simulink model "six_plus_six_AcmsteeringV09_main"  (R2014a)
settings: Solver=FixedStepDiscrete  StartTime=0.0  StopTime=10.0  FixedStep=0.0005  RelTol=1e-3
InitFcn:
  | Veh_Par_wxt
values from neighbouring files (symbols this model uses):
  acc_spdctl = [0 100]    [Veh_Par_wxt.m]
  ag_thr = ecucoder_cal(ag_thr)    [Veh_Par_wxt.m]
  B = 1.8    [Veh_Par_wxt.m]
  bra_em = 100    [Veh_Par_wxt.m]
  bra_pre_gz2 = 100/3    (= 33.3333333333)    [Veh_Par_wxt.m]
  bra_pre_gz34 = 10/3    (= 3.33333333333)    [Veh_Par_wxt.m]
  bra_pre_yd = 10/2    (= 5)    [Veh_Par_wxt.m]
  brakepre_dem_data = [0 1 2 3 4 5 6 7 8 9 10]    [Veh_Par_wxt.m]
  brakeTrq_dem_data = [0 125 251 376 502 627 753 878 1004 1129 1255]    [Veh_Par_wxt.m]
  bratrq_max = 4*1255    (= 5020)    [Veh_Par_wxt.m]
  eff_tran = 0.9    [Veh_Par_wxt.m]
  ESP_switch = ecucoder_cal(ESP_switch)    [Veh_Par_wxt.m]
  G = Mass*g    (= 15696)    [Veh_Par_wxt.m]
  kd1 = ecucoder_cal(kd1)    [Veh_Par_wxt.m]
  kd2 = 0    [Veh_Par_wxt.m]
  ki1 = ecucoder_cal(ki1)    [Veh_Par_wxt.m]
  ki2 = 1    [Veh_Par_wxt.m]
  kp1 = ecucoder_cal(kp1)    [Veh_Par_wxt.m]
  kp2 = 300    [Veh_Par_wxt.m]
  L = L1+L2    (= 2.9)    [Veh_Par_wxt.m]
  premax = 100    [Veh_Par_wxt.m]
  Radius = 0.4572/2    (= 0.2286)    [Veh_Par_wxt.m]
  RC_switch = ecucoder_cal(RC_switch)    [Veh_Par_wxt.m]
  s_opt_yi = 0.15    [Veh_Par_wxt.m]
  s_opt_zhuan = 0.8    [Veh_Par_wxt.m]
  s_opt_zhuan_add = 0.05    [Veh_Par_wxt.m]
  s_opt_zhuan_table = [0.8 0.8 0.3 0.3]    [Veh_Par_wxt.m]
  spd_map_mot = [0 499.85 999.79 1500 2000 2500 3000 3500 4000 4500 4999.8 5999.8]    [Veh_Par_wxt.m]
  spd_spdctl = [0 500]    [Veh_Par_wxt.m]
  speed_thr_park = 5/3.6/Radius*tras_ratio*30/pi    (= 464.143899364)    [Veh_Par_wxt.m]
  TCS_switch = ecucoder_cal(TCS_switch)    [Veh_Par_wxt.m]
  tras_ratio = 8    [Veh_Par_wxt.m]
  trq_map_mot = [70.5 70.012 71.154 65.797 53.917 45.159 38.073 32.685 27.48 17.133 14.949 10.07]    [Veh_Par_wxt.m]
  trqmax_yd = 70.5    [Veh_Par_wxt.m]
  trqmax_zx = 70.5    [Veh_Par_wxt.m]
  trqmaxneg = -70.5    [Veh_Par_wxt.m]
  v_gain = 0.9    [Veh_Par_wxt.m]
  v_table = [0 5 20 100]    [Veh_Par_wxt.m]
  v_thr_park = 5    [Veh_Par_wxt.m]
  zhidong_bianmazhi = [-140000 750000]    [Veh_Par_wxt.m]
  zhidong_down = -140000    [Veh_Par_wxt.m]
  zhidong_up = 750000    [Veh_Par_wxt.m]
  zhidong_youmen = [0 100]    [Veh_Par_wxt.m]
  zhuanxiang_bianmazhi = [-400000 0 400000]    [Veh_Par_wxt.m]
  zhuanxiang_down = -400000    [Veh_Par_wxt.m]
  zhuanxiang_up = 400000    [Veh_Par_wxt.m]
  zhuanxiang_youmen = [-100 0 100]    [Veh_Par_wxt.m]
undefined symbols (not defined in the file or in its folder): ecucoder_acal, guzhang_lf, guzhang_lm, guzhang_lr, guzhang_rf, guzhang_rm, guzhang_rr, myFIS
libraries: simulink x979, ec5744lib x59, fuzblock x2
(part 8 of 26)

== system six_plus_six_AcmsteeringV09_main/Data_input/MCU0_4/MCU0 ==
  input : Inport
  Enable : EnablePort
  Demux : Demux  Outputs=8
  MCU0_ControlMode_Ad : Sum
  MCU0_ControlMode_Convert : DataTypeConversion  OutDataTypeStr=uint32
  MCU0_ControlMode_F : Gain
  MCU0_ControlMode_L : simulink/Logic and Bit Operations/Bitwise Operator  logicop=AND  UseBitMask=on  BitMask=4  BitMaskRealWorld=Stored Integer
  MCU0_ControlMode_O : Constant  Value=0  OutDataTypeStr=single
  MCU0_ControlMode_S : ArithShift  BitShiftNumber=2
  MCU0_ControlMode_Sub : Subsystem
  MCU0_ControlMode_sat : Saturate  UpperLimit=1  LowerLimit=0
  MCU0_ControlModecv : DataTypeConversion
  MCU0_EmergShutDown_Ad : Sum
  MCU0_EmergShutDown_Convert : DataTypeConversion  OutDataTypeStr=uint32
  MCU0_EmergShutDown_F : Gain
  MCU0_EmergShutDown_L : simulink/Logic and Bit Operations/Bitwise Operator  logicop=AND  UseBitMask=on  BitMask=128  BitMaskRealWorld=Stored Integer
  MCU0_EmergShutDown_O : Constant  Value=0  OutDataTypeStr=single
  MCU0_EmergShutDown_S : ArithShift  BitShiftNumber=7
  MCU0_EmergShutDown_Sub : Subsystem
  MCU0_EmergShutDown_sat : Saturate  UpperLimit=1  LowerLimit=0
  MCU0_EmergShutDowncv : DataTypeConversion
  MCU0_GearStatus_Ad : Sum
  MCU0_GearStatus_Convert : DataTypeConversion  OutDataTypeStr=uint32
  MCU0_GearStatus_F : Gain
  MCU0_GearStatus_L : simulink/Logic and Bit Operations/Bitwise Operator  logicop=AND  UseBitMask=on  BitMask=24  BitMaskRealWorld=Stored Integer
  MCU0_GearStatus_O : Constant  Value=0  OutDataTypeStr=single
  MCU0_GearStatus_S : ArithShift  BitShiftNumber=3
  MCU0_GearStatus_Sub : Subsystem
  MCU0_GearStatus_sat : Saturate  UpperLimit=3  LowerLimit=0
  MCU0_GearStatuscv : DataTypeConversion
  MCU0_HighVol_Ad : Sum
  MCU0_HighVol_Convert : DataTypeConversion  OutDataTypeStr=uint32
  MCU0_HighVol_F : Gain
  MCU0_HighVol_L : simulink/Logic and Bit Operations/Bitwise Operator  logicop=AND  UseBitMask=on  BitMask=32  BitMaskRealWorld=Stored Integer
  MCU0_HighVol_O : Constant  Value=0  OutDataTypeStr=single
  MCU0_HighVol_S : ArithShift  BitShiftNumber=5
  MCU0_HighVol_Sub : Subsystem
  MCU0_HighVol_sat : Saturate  UpperLimit=1  LowerLimit=0
  MCU0_HighVolcv : DataTypeConversion
  MCU0_LiftCnt_Ad : Sum
  MCU0_LiftCnt_Convert : DataTypeConversion  OutDataTypeStr=uint32
  MCU0_LiftCnt_F : Gain
  MCU0_LiftCnt_L : simulink/Logic and Bit Operations/Bitwise Operator  logicop=AND  UseBitMask=on  BitMask=255  BitMaskRealWorld=Stored Integer
  MCU0_LiftCnt_O : Constant  Value=0  OutDataTypeStr=single
  MCU0_LiftCnt_S : ArithShift
  MCU0_LiftCnt_Sub : Subsystem
  MCU0_LiftCnt_sat : Saturate  UpperLimit=255  LowerLimit=0
  MCU0_LiftCntcv : DataTypeConversion
  MCU0_ShutDowAllow_Ad : Sum
  MCU0_ShutDowAllow_Convert : DataTypeConversion  OutDataTypeStr=uint32
  MCU0_ShutDowAllow_F : Gain
  MCU0_ShutDowAllow_L : simulink/Logic and Bit Operations/Bitwise Operator  logicop=AND  UseBitMask=on  BitMask=64  BitMaskRealWorld=Stored Integer
  MCU0_ShutDowAllow_O : Constant  Value=0  OutDataTypeStr=single
  MCU0_ShutDowAllow_S : ArithShift  BitShiftNumber=6
  MCU0_ShutDowAllow_Sub : Subsystem
  MCU0_ShutDowAllow_sat : Saturate  UpperLimit=1  LowerLimit=0
  MCU0_ShutDowAllowcv : DataTypeConversion
  MCU0_SpeedFdk_Ad : Sum
  MCU0_SpeedFdk_Convert : DataTypeConversion  OutDataTypeStr=uint32
  MCU0_SpeedFdk_F : Gain
  MCU0_SpeedFdk_L : simulink/Logic and Bit Operations/Bitwise Operator  logicop=AND  UseBitMask=on  BitMask=65535  BitMaskRealWorld=Stored Integer
  MCU0_SpeedFdk_O : Constant  Value=-10000  OutDataTypeStr=single
  MCU0_SpeedFdk_S : ArithShift
  MCU0_SpeedFdk_Sub : Subsystem
  MCU0_SpeedFdk_sat : Saturate  UpperLimit=10000  LowerLimit=-10000
  MCU0_SpeedFdkcv : DataTypeConversion
  MCU0_SpeedFdkinput2_Ad : Sum
  MCU0_SpeedFdkinput2_C : Constant  Value=256
  MCU0_SpeedFdkinput2_P : Product
  MCU0_TorqueFdk_Ad : Sum
  MCU0_TorqueFdk_Convert : DataTypeConversion  OutDataTypeStr=uint32
  MCU0_TorqueFdk_F : Gain  Gain=0.1
  MCU0_TorqueFdk_L : simulink/Logic and Bit Operations/Bitwise Operator  logicop=AND  UseBitMask=on  BitMask=65535  BitMaskRealWorld=Stored Integer
  MCU0_TorqueFdk_O : Constant  Value=-1000  OutDataTypeStr=single
  MCU0_TorqueFdk_S : ArithShift
  MCU0_TorqueFdk_Sub : Subsystem
  MCU0_TorqueFdk_sat : Saturate  UpperLimit=1000  LowerLimit=-1000
  MCU0_TorqueFdkcv : DataTypeConversion
  MCU0_TorqueFdkinput4_Ad : Sum
  MCU0_TorqueFdkinput4_C : Constant  Value=256
  MCU0_TorqueFdkinput4_P : Product
  MCU0_TorqueMax_Ad : Sum
  MCU0_TorqueMax_Convert : DataTypeConversion  OutDataTypeStr=uint32
  MCU0_TorqueMax_F : Gain  Gain=0.1
  MCU0_TorqueMax_L : simulink/Logic and Bit Operations/Bitwise Operator  logicop=AND  UseBitMask=on  BitMask=65535  BitMaskRealWorld=Stored Integer
  MCU0_TorqueMax_O : Constant  Value=-1000  OutDataTypeStr=single
  MCU0_TorqueMax_S : ArithShift
  MCU0_TorqueMax_Sub : Subsystem
  MCU0_TorqueMax_sat : Saturate  UpperLimit=1000  LowerLimit=-1000
  MCU0_TorqueMaxcv : DataTypeConversion
  MCU0_TorqueMaxinput6_Ad : Sum
  MCU0_TorqueMaxinput6_C : Constant  Value=256
  MCU0_TorqueMaxinput6_P : Product
  MCU0_WorkStatus_Ad : Sum
  MCU0_WorkStatus_Convert : DataTypeConversion  OutDataTypeStr=uint32
  MCU0_WorkStatus_F : Gain
  MCU0_WorkStatus_L : simulink/Logic and Bit Operations/Bitwise Operator  logicop=AND  UseBitMask=on  BitMask=3  BitMaskRealWorld=Stored Integer
  MCU0_WorkStatus_O : Constant  Value=0  OutDataTypeStr=single
  MCU0_WorkStatus_S : ArithShift
  MCU0_WorkStatus_Sub : Subsystem
  MCU0_WorkStatus_sat : Saturate  UpperLimit=3  LowerLimit=0
  MCU0_WorkStatuscv : DataTypeConversion
  MCU0_TorqueMax_Out : Outport
  MCU0_EmergShutDown_Out : Outport  Port=2
  MCU0_ShutDowAllow_Out : Outport  Port=3
  MCU0_HighVol_Out : Outport  Port=4
  MCU0_LiftCnt_Out : Outport  Port=5
  MCU0_TorqueFdk_Out : Outport  Port=6
  MCU0_SpeedFdk_Out : Outport  Port=7
  MCU0_GearStatus_Out : Outport  Port=8
  MCU0_ControlMode_Out : Outport  Port=9
  MCU0_WorkStatus_Out : Outport  Port=10
  wires:
  MCU0_TorqueMax_F/1 -> MCU0_TorqueMax_Ad/1
  MCU0_TorqueMax_O/1 -> MCU0_TorqueMax_Ad/2
  MCU0_TorqueMax_Ad/1 -> MCU0_TorqueMax_sat/1
  MCU0_TorqueMax_sat/1 -> MCU0_TorqueMax_Out/1
  Demux/6 -> MCU0_TorqueMaxinput6_P/1
  MCU0_TorqueMaxinput6_C/1 -> MCU0_TorqueMaxinput6_P/2
  MCU0_TorqueMaxinput6_P/1 -> MCU0_TorqueMaxinput6_Ad/1
  Demux/7 -> MCU0_TorqueMaxinput6_Ad/2
  MCU0_TorqueMaxinput6_Ad/1 -> MCU0_TorqueMax_Sub/1(In1)
  MCU0_TorqueMax_Sub/1(Out1) -> MCU0_TorqueMax_Convert/1
  MCU0_TorqueMax_Convert/1 -> MCU0_TorqueMax_L/1
  MCU0_TorqueMax_L/1 -> MCU0_TorqueMax_S/1
  MCU0_TorqueMax_S/1 -> MCU0_TorqueMaxcv/1
  MCU0_TorqueMaxcv/1 -> MCU0_TorqueMax_F/1
  MCU0_EmergShutDown_F/1 -> MCU0_EmergShutDown_Ad/1
  MCU0_EmergShutDown_O/1 -> MCU0_EmergShutDown_Ad/2
  MCU0_EmergShutDown_Ad/1 -> MCU0_EmergShutDown_sat/1
  MCU0_EmergShutDown_sat/1 -> MCU0_EmergShutDown_Out/1
  Demux/1 -> MCU0_ControlMode_Sub/1(In1), MCU0_WorkStatus_Sub/1(In1), MCU0_GearStatus_Sub/1(In1), MCU0_HighVol_Sub/1(In1), MCU0_ShutDowAllow_Sub/1(In1), MCU0_EmergShutDown_Sub/1(In1)
  MCU0_EmergShutDown_Sub/1(Out1) -> MCU0_EmergShutDown_Convert/1
  MCU0_EmergShutDown_Convert/1 -> MCU0_EmergShutDown_L/1
  MCU0_EmergShutDown_L/1 -> MCU0_EmergShutDown_S/1
  MCU0_EmergShutDown_S/1 -> MCU0_EmergShutDowncv/1
  MCU0_EmergShutDowncv/1 -> MCU0_EmergShutDown_F/1
  MCU0_ShutDowAllow_F/1 -> MCU0_ShutDowAllow_Ad/1
  MCU0_ShutDowAllow_O/1 -> MCU0_ShutDowAllow_Ad/2
  MCU0_ShutDowAllow_Ad/1 -> MCU0_ShutDowAllow_sat/1
  MCU0_ShutDowAllow_sat/1 -> MCU0_ShutDowAllow_Out/1
  MCU0_ShutDowAllow_Sub/1(Out1) -> MCU0_ShutDowAllow_Convert/1
  MCU0_ShutDowAllow_Convert/1 -> MCU0_ShutDowAllow_L/1
  MCU0_ShutDowAllow_L/1 -> MCU0_ShutDowAllow_S/1
  MCU0_ShutDowAllow_S/1 -> MCU0_ShutDowAllowcv/1
  MCU0_ShutDowAllowcv/1 -> MCU0_ShutDowAllow_F/1
  MCU0_HighVol_F/1 -> MCU0_HighVol_Ad/1
  MCU0_HighVol_O/1 -> MCU0_HighVol_Ad/2
  MCU0_HighVol_Ad/1 -> MCU0_HighVol_sat/1
  MCU0_HighVol_sat/1 -> MCU0_HighVol_Out/1
  MCU0_HighVol_Sub/1(Out1) -> MCU0_HighVol_Convert/1
  MCU0_HighVol_Convert/1 -> MCU0_HighVol_L/1
  MCU0_HighVol_L/1 -> MCU0_HighVol_S/1
  MCU0_HighVol_S/1 -> MCU0_HighVolcv/1
  MCU0_HighVolcv/1 -> MCU0_HighVol_F/1
  MCU0_LiftCnt_F/1 -> MCU0_LiftCnt_Ad/1
  MCU0_LiftCnt_O/1 -> MCU0_LiftCnt_Ad/2
  MCU0_LiftCnt_Ad/1 -> MCU0_LiftCnt_sat/1
  MCU0_LiftCnt_sat/1 -> MCU0_LiftCnt_Out/1
  Demux/8 -> MCU0_LiftCnt_Sub/1(In1)
  MCU0_LiftCnt_Sub/1(Out1) -> MCU0_LiftCnt_Convert/1
  MCU0_LiftCnt_Convert/1 -> MCU0_LiftCnt_L/1
  MCU0_LiftCnt_L/1 -> MCU0_LiftCnt_S/1
  MCU0_LiftCnt_S/1 -> MCU0_LiftCntcv/1
  MCU0_LiftCntcv/1 -> MCU0_LiftCnt_F/1
  MCU0_TorqueFdk_F/1 -> MCU0_TorqueFdk_Ad/1
  MCU0_TorqueFdk_O/1 -> MCU0_TorqueFdk_Ad/2
  MCU0_TorqueFdk_Ad/1 -> MCU0_TorqueFdk_sat/1
  MCU0_TorqueFdk_sat/1 -> MCU0_TorqueFdk_Out/1
  Demux/4 -> MCU0_TorqueFdkinput4_P/1
  MCU0_TorqueFdkinput4_C/1 -> MCU0_TorqueFdkinput4_P/2
  MCU0_TorqueFdkinput4_P/1 -> MCU0_TorqueFdkinput4_Ad/1
  Demux/5 -> MCU0_TorqueFdkinput4_Ad/2
  MCU0_TorqueFdkinput4_Ad/1 -> MCU0_TorqueFdk_Sub/1(In1)
  MCU0_TorqueFdk_Sub/1(Out1) -> MCU0_TorqueFdk_Convert/1
  MCU0_TorqueFdk_Convert/1 -> MCU0_TorqueFdk_L/1
  MCU0_TorqueFdk_L/1 -> MCU0_TorqueFdk_S/1
  MCU0_TorqueFdk_S/1 -> MCU0_TorqueFdkcv/1
  MCU0_TorqueFdkcv/1 -> MCU0_TorqueFdk_F/1
  MCU0_SpeedFdk_F/1 -> MCU0_SpeedFdk_Ad/1
  MCU0_SpeedFdk_O/1 -> MCU0_SpeedFdk_Ad/2
  MCU0_SpeedFdk_Ad/1 -> MCU0_SpeedFdk_sat/1
  MCU0_SpeedFdk_sat/1 -> MCU0_SpeedFdk_Out/1
  Demux/2 -> MCU0_SpeedFdkinput2_P/1
  MCU0_SpeedFdkinput2_C/1 -> MCU0_SpeedFdkinput2_P/2
  MCU0_SpeedFdkinput2_P/1 -> MCU0_SpeedFdkinput2_Ad/1
  Demux/3 -> MCU0_SpeedFdkinput2_Ad/2
  MCU0_SpeedFdkinput2_Ad/1 -> MCU0_SpeedFdk_Sub/1(In1)
  MCU0_SpeedFdk_Sub/1(Out1) -> MCU0_SpeedFdk_Convert/1
  MCU0_SpeedFdk_Convert/1 -> MCU0_SpeedFdk_L/1
  MCU0_SpeedFdk_L/1 -> MCU0_SpeedFdk_S/1
  MCU0_SpeedFdk_S/1 -> MCU0_SpeedFdkcv/1
  MCU0_SpeedFdkcv/1 -> MCU0_SpeedFdk_F/1
  MCU0_GearStatus_F/1 -> MCU0_GearStatus_Ad/1
  MCU0_GearStatus_O/1 -> MCU0_GearStatus_Ad/2
  MCU0_GearStatus_Ad/1 -> MCU0_GearStatus_sat/1
  MCU0_GearStatus_sat/1 -> MCU0_GearStatus_Out/1
  MCU0_GearStatus_Sub/1(Out1) -> MCU0_GearStatus_Convert/1
  MCU0_GearStatus_Convert/1 -> MCU0_GearStatus_L/1
  MCU0_GearStatus_L/1 -> MCU0_GearStatus_S/1
  MCU0_GearStatus_S/1 -> MCU0_GearStatuscv/1
  MCU0_GearStatuscv/1 -> MCU0_GearStatus_F/1
  MCU0_ControlMode_F/1 -> MCU0_ControlMode_Ad/1
  MCU0_ControlMode_O/1 -> MCU0_ControlMode_Ad/2
  MCU0_ControlMode_Ad/1 -> MCU0_ControlMode_sat/1
  MCU0_ControlMode_sat/1 -> MCU0_ControlMode_Out/1
  MCU0_ControlMode_Sub/1(Out1) -> MCU0_ControlMode_Convert/1
  MCU0_ControlMode_Convert/1 -> MCU0_ControlMode_L/1
  MCU0_ControlMode_L/1 -> MCU0_ControlMode_S/1
  MCU0_ControlMode_S/1 -> MCU0_ControlModecv/1
  MCU0_ControlModecv/1 -> MCU0_ControlMode_F/1
  MCU0_WorkStatus_F/1 -> MCU0_WorkStatus_Ad/1
  MCU0_WorkStatus_O/1 -> MCU0_WorkStatus_Ad/2
  MCU0_WorkStatus_Ad/1 -> MCU0_WorkStatus_sat/1
  MCU0_WorkStatus_sat/1 -> MCU0_WorkStatus_Out/1
  MCU0_WorkStatus_Sub/1(Out1) -> MCU0_WorkStatus_Convert/1
  MCU0_WorkStatus_Convert/1 -> MCU0_WorkStatus_L/1
  MCU0_WorkStatus_L/1 -> MCU0_WorkStatus_S/1
  MCU0_WorkStatus_S/1 -> MCU0_WorkStatuscv/1
  MCU0_WorkStatuscv/1 -> MCU0_WorkStatus_F/1
  input/1 -> Demux/1

== matlab function six_plus_six_AcmsteeringV09_main/MainControl/mode_control/forward/forward/Brake/HeartBeat5 ==
  data: life_pre input; life output
function life = fcn(life_pre)
%#codegen
life=single(life_pre+1);
if life>255
    life=single(0);
end
end

== matlab function six_plus_six_AcmsteeringV09_main/MainControl/mode_control/neutral/neutral/HeartBeat2 ==
  data: life_pre input; life output
function life = fcn(life_pre)
%#codegen
life=single(life_pre+1);
if life>255
    life=single(0);
end
end

== matlab function six_plus_six_AcmsteeringV09_main/MainControl/mode_control/backward/backward/Brake/HeartBeat4 ==
  data: life_pre input; life output
function life = fcn(life_pre)
%#codegen
life=single(life_pre+1);
if life>255
    life=single(0);
end
end

== matlab function six_plus_six_AcmsteeringV09_main/MainControl/mode_control/backward/backward/Drive/目标转向力矩确定模块/MATLAB Function1 ==
  data: v_act input; Rturn_min_ag output; ag_thr input
 function Rturn_min_ag = fcn(v_act,ag_thr)
%#codegen

    Rturn_min_ag=single((v_act/3.6)^2/ag_thr);
end

== matlab function six_plus_six_AcmsteeringV09_main/MainControl/mode_control/backward/backward/Drive/驱动防滑控制TCS/直行TCS/直行/HeartBeat ==
  data: life_pre input; life output
function life = fcn(life_pre)
%#codegen
life=single(life_pre+1);
if life>255
    life=single(0);
end
end

== matlab function six_plus_six_AcmsteeringV09_main/MainControl/mode_control/backward/backward/Drive/驱动防滑控制TCS/直行TCS/直行/HeartBeat2 ==
  data: life_pre input; life output
function life = fcn(life_pre)
%#codegen
life=single(life_pre+1);
if life>255
    life=single(0);
end
end

== matlab function six_plus_six_AcmsteeringV09_main/MainControl/mode_control/backward/backward/MATLAB Function ==
  data: acc_dem input; y output; brake_dem input; HAC input
function y = fcn(acc_dem,brake_dem,HAC)
%#codegen
if HAC==1
    if acc_dem<0
        y=int8(0);
    else
        y=int8(1);
    end
else
    if brake_dem==0
        y=int8(0);
    else
        y=int8(1);
    end
end
end

== matlab function six_plus_six_AcmsteeringV09_main/MainControl/mode_control/emergency_stop/emergency_stop/HeartBeat1 ==
  data: life_pre input; life output
function life = fcn(life_pre)
%#codegen
life=single(life_pre+1);
if life>255
    life=single(0);
end
end

== matlab function six_plus_six_AcmsteeringV09_main/Data_input/1/Enabled
Subsystem/MATLAB Function1 ==
  data: current_in input; current_out output
function current_out = motec_current(current_in)
    if current_in>32768
        current_out=current_in-65535;
    else
        current_out=current_in;
    end
end

== matlab function six_plus_six_AcmsteeringV09_main/MainControl/mode_control/forward/forward/Drive/驱动防滑控制TCS/直行TCS/直行/MATLAB Function6 ==
  data: s_act_rm input; flag_rm output; s_opt_zhuan input; s_opt_zhuan_add input; flag_rm_pre input int8
function flag_rm = fcn(s_act_rm,s_opt_zhuan,s_opt_zhuan_add,flag_rm_pre)
%#codegen
if s_act_rm>s_opt_zhuan+s_opt_zhuan_add
    flag_rm=int8(1);
elseif s_act_rm<s_opt_zhuan
    flag_rm =int8(0);
else
    flag_rm=int8(flag_rm_pre);
end
end

== matlab function six_plus_six_AcmsteeringV09_main/Data_input/4/Enabled Subsystem/MATLAB Function ==
  data: data1 input; y output; data2 input; data3 input; data4 input
function y = fcn(data1,data2,data3,data4)
%#codegen
y1=data4*256^3+data3*256^2+data2*256+data1;
y=typecast(uint32(y1),'single');
end
% y = u;

== matlab function six_plus_six_AcmsteeringV09_main/Data_input/6/Enabled
Subsystem/MATLAB Function1 ==
  data: data1 input; y output; data2 input; data3 input; data4 input
function y = fcn(data1,data2,data3,data4)
%#codegen
y1=data4*256^3+data3*256^2+data2*256+data1;
y=typecast(uint32(y1),'single');
end
% y = u;

== matlab function six_plus_six_AcmsteeringV09_main/Data_input/10/Enabled Subsystem/MATLAB Function ==
  data: data1 input; y output; data2 input; data3 input; data4 input
function y = fcn(data1,data2,data3,data4)
%#codegen
y1=data4*256^3+data3*256^2+data2*256+data1;
y=typecast(uint32(y1),'single');
end
% y = u;

== matlab function six_plus_six_AcmsteeringV09_main/MainControl/mode_control/forward/forward/Drive/MATLAB Function ==
  data: acc_y input; y output; ag_thr input
function y = fcn(acc_y,ag_thr)
%#codegen
if abs(acc_y)>=ag_thr
    y=int8(0);
else 
    y=int8(1);
end
end

== matlab function six_plus_six_AcmsteeringV09_main/MainControl/mode_control/forward/forward/Drive/驱动防滑控制TCS/直行TCS/直行/MATLAB Function5 ==
  data: TCS_switch input; flag_lf1 output; flag_lm1 output; flag_lf input; flag_lm input; flag_lr input; flag_lr1 output; flag_rf input; flag_rm input; flag_rr input; flag_rf1 output; flag_rm1 output; flag_rr1 output
 function [flag_lf1,flag_lm1,flag_lr1,flag_rf1,flag_rm1,flag_rr1] = fcn(TCS_switch,flag_lf,flag_lm,flag_lr,flag_rf,flag_rm,flag_rr)
%#codegen
if TCS_switch==0
    flag_lf1=single(0);
    flag_lm1=single(0);
    flag_lr1=single(0);
    flag_rf1=single(0);
    flag_rm1=single(0);
    flag_rr1=single(0);
else
    flag_lf1=single(flag_lf);
    flag_lm1=single(flag_lm);
    flag_lr1=single(flag_lr);
    flag_rf1=single(flag_rf);
    flag_rm1=single(flag_rm);
    flag_rr1=single(flag_rr);
end
end

== system six_plus_six_AcmsteeringV09_main/Data_input/MCU0_5/MCU0 ==
  input : Inport
  Enable : EnablePort
  Demux : Demux  Outputs=8
  MCU0_ControlMode_Ad : Sum
  MCU0_ControlMode_Convert : DataTypeConversion  OutDataTypeStr=uint32
  MCU0_ControlMode_F : Gain
  MCU0_ControlMode_L : simulink/Logic and Bit Operations/Bitwise Operator  logicop=AND  UseBitMask=on  BitMask=4  BitMaskRealWorld=Stored Integer
  MCU0_ControlMode_O : Constant  Value=0  OutDataTypeStr=single
  MCU0_ControlMode_S : ArithShift  BitShiftNumber=2
  MCU0_ControlMode_Sub : Subsystem
  MCU0_ControlMode_sat : Saturate  UpperLimit=1  LowerLimit=0
  MCU0_ControlModecv : DataTypeConversion
  MCU0_EmergShutDown_Ad : Sum
  MCU0_EmergShutDown_Convert : DataTypeConversion  OutDataTypeStr=uint32
  MCU0_EmergShutDown_F : Gain
  MCU0_EmergShutDown_L : simulink/Logic and Bit Operations/Bitwise Operator  logicop=AND  UseBitMask=on  BitMask=128  BitMaskRealWorld=Stored Integer
  MCU0_EmergShutDown_O : Constant  Value=0  OutDataTypeStr=single
  MCU0_EmergShutDown_S : ArithShift  BitShiftNumber=7
  MCU0_EmergShutDown_Sub : Subsystem
  MCU0_EmergShutDown_sat : Saturate  UpperLimit=1  LowerLimit=0
  MCU0_EmergShutDowncv : DataTypeConversion
  MCU0_GearStatus_Ad : Sum
  MCU0_GearStatus_Convert : DataTypeConversion  OutDataTypeStr=uint32
  MCU0_GearStatus_F : Gain
  MCU0_GearStatus_L : simulink/Logic and Bit Operations/Bitwise Operator  logicop=AND  UseBitMask=on  BitMask=24  BitMaskRealWorld=Stored Integer
  MCU0_GearStatus_O : Constant  Value=0  OutDataTypeStr=single
  MCU0_GearStatus_S : ArithShift  BitShiftNumber=3
  MCU0_GearStatus_Sub : Subsystem
  MCU0_GearStatus_sat : Saturate  UpperLimit=3  LowerLimit=0
  MCU0_GearStatuscv : DataTypeConversion
  MCU0_HighVol_Ad : Sum
  MCU0_HighVol_Convert : DataTypeConversion  OutDataTypeStr=uint32
  MCU0_HighVol_F : Gain
  MCU0_HighVol_L : simulink/Logic and Bit Operations/Bitwise Operator  logicop=AND  UseBitMask=on  BitMask=32  BitMaskRealWorld=Stored Integer
  MCU0_HighVol_O : Constant  Value=0  OutDataTypeStr=single
  MCU0_HighVol_S : ArithShift  BitShiftNumber=5
  MCU0_HighVol_Sub : Subsystem
  MCU0_HighVol_sat : Saturate  UpperLimit=1  LowerLimit=0
  MCU0_HighVolcv : DataTypeConversion
  MCU0_LiftCnt_Ad : Sum
  MCU0_LiftCnt_Convert : DataTypeConversion  OutDataTypeStr=uint32
  MCU0_LiftCnt_F : Gain
  MCU0_LiftCnt_L : simulink/Logic and Bit Operations/Bitwise Operator  logicop=AND  UseBitMask=on  BitMask=255  BitMaskRealWorld=Stored Integer
  MCU0_LiftCnt_O : Constant  Value=0  OutDataTypeStr=single
  MCU0_LiftCnt_S : ArithShift
  MCU0_LiftCnt_Sub : Subsystem
  MCU0_LiftCnt_sat : Saturate  UpperLimit=255  LowerLimit=0
  MCU0_LiftCntcv : DataTypeConversion
  MCU0_ShutDowAllow_Ad : Sum
  MCU0_ShutDowAllow_Convert : DataTypeConversion  OutDataTypeStr=uint32
  MCU0_ShutDowAllow_F : Gain
  MCU0_ShutDowAllow_L : simulink/Logic and Bit Operations/Bitwise Operator  logicop=AND  UseBitMask=on  BitMask=64  BitMaskRealWorld=Stored Integer
  MCU0_ShutDowAllow_O : Constant  Value=0  OutDataTypeStr=single
  MCU0_ShutDowAllow_S : ArithShift  BitShiftNumber=6
  MCU0_ShutDowAllow_Sub : Subsystem
  MCU0_ShutDowAllow_sat : Saturate  UpperLimit=1  LowerLimit=0
  MCU0_ShutDowAllowcv : DataTypeConversion
  MCU0_SpeedFdk_Ad : Sum
  MCU0_SpeedFdk_Convert : DataTypeConversion  OutDataTypeStr=uint32
  MCU0_SpeedFdk_F : Gain
  MCU0_SpeedFdk_L : simulink/Logic and Bit Operations/Bitwise Operator  logicop=AND  UseBitMask=on  BitMask=65535  BitMaskRealWorld=Stored Integer
  MCU0_SpeedFdk_O : Constant  Value=-10000  OutDataTypeStr=single
  MCU0_SpeedFdk_S : ArithShift
  MCU0_SpeedFdk_Sub : Subsystem
  MCU0_SpeedFdk_sat : Saturate  UpperLimit=10000  LowerLimit=-10000
  MCU0_SpeedFdkcv : DataTypeConversion
  MCU0_SpeedFdkinput2_Ad : Sum
  MCU0_SpeedFdkinput2_C : Constant  Value=256
  MCU0_SpeedFdkinput2_P : Product
  MCU0_TorqueFdk_Ad : Sum
  MCU0_TorqueFdk_Convert : DataTypeConversion  OutDataTypeStr=uint32
  MCU0_TorqueFdk_F : Gain  Gain=0.1
  MCU0_TorqueFdk_L : simulink/Logic and Bit Operations/Bitwise Operator  logicop=AND  UseBitMask=on  BitMask=65535  BitMaskRealWorld=Stored Integer
  MCU0_TorqueFdk_O : Constant  Value=-1000  OutDataTypeStr=single
  MCU0_TorqueFdk_S : ArithShift
  MCU0_TorqueFdk_Sub : Subsystem
  MCU0_TorqueFdk_sat : Saturate  UpperLimit=1000  LowerLimit=-1000
  MCU0_TorqueFdkcv : DataTypeConversion
  MCU0_TorqueFdkinput4_Ad : Sum
  MCU0_TorqueFdkinput4_C : Constant  Value=256
  MCU0_TorqueFdkinput4_P : Product
  MCU0_TorqueMax_Ad : Sum
  MCU0_TorqueMax_Convert : DataTypeConversion  OutDataTypeStr=uint32
  MCU0_TorqueMax_F : Gain  Gain=0.1
  MCU0_TorqueMax_L : simulink/Logic and Bit Operations/Bitwise Operator  logicop=AND  UseBitMask=on  BitMask=65535  BitMaskRealWorld=Stored Integer
  MCU0_TorqueMax_O : Constant  Value=-1000  OutDataTypeStr=single
  MCU0_TorqueMax_S : ArithShift
  MCU0_TorqueMax_Sub : Subsystem
  MCU0_TorqueMax_sat : Saturate  UpperLimit=1000  LowerLimit=-1000
  MCU0_TorqueMaxcv : DataTypeConversion
  MCU0_TorqueMaxinput6_Ad : Sum
  MCU0_TorqueMaxinput6_C : Constant  Value=256
  MCU0_TorqueMaxinput6_P : Product
  MCU0_WorkStatus_Ad : Sum
  MCU0_WorkStatus_Convert : DataTypeConversion  OutDataTypeStr=uint32
  MCU0_WorkStatus_F : Gain
  MCU0_WorkStatus_L : simulink/Logic and Bit Operations/Bitwise Operator  logicop=AND  UseBitMask=on  BitMask=3  BitMaskRealWorld=Stored Integer
  MCU0_WorkStatus_O : Constant  Value=0  OutDataTypeStr=single
  MCU0_WorkStatus_S : ArithShift
  MCU0_WorkStatus_Sub : Subsystem
  MCU0_WorkStatus_sat : Saturate  UpperLimit=3  LowerLimit=0
  MCU0_WorkStatuscv : DataTypeConversion
  MCU0_TorqueMax_Out : Outport
  MCU0_EmergShutDown_Out : Outport  Port=2
  MCU0_ShutDowAllow_Out : Outport  Port=3
  MCU0_HighVol_Out : Outport  Port=4
  MCU0_LiftCnt_Out : Outport  Port=5
  MCU0_TorqueFdk_Out : Outport  Port=6
  MCU0_SpeedFdk_Out : Outport  Port=7
  MCU0_GearStatus_Out : Outport  Port=8
  MCU0_ControlMode_Out : Outport  Port=9
  MCU0_WorkStatus_Out : Outport  Port=10
  wires:
  MCU0_TorqueMax_F/1 -> MCU0_TorqueMax_Ad/1
  MCU0_TorqueMax_O/1 -> MCU0_TorqueMax_Ad/2
  MCU0_TorqueMax_Ad/1 -> MCU0_TorqueMax_sat/1
  MCU0_TorqueMax_sat/1 -> MCU0_TorqueMax_Out/1
  Demux/6 -> MCU0_TorqueMaxinput6_P/1
  MCU0_TorqueMaxinput6_C/1 -> MCU0_TorqueMaxinput6_P/2
  MCU0_TorqueMaxinput6_P/1 -> MCU0_TorqueMaxinput6_Ad/1
  Demux/7 -> MCU0_TorqueMaxinput6_Ad/2
  MCU0_TorqueMaxinput6_Ad/1 -> MCU0_TorqueMax_Sub/1(In1)
  MCU0_TorqueMax_Sub/1(Out1) -> MCU0_TorqueMax_Convert/1
  MCU0_TorqueMax_Convert/1 -> MCU0_TorqueMax_L/1
  MCU0_TorqueMax_L/1 -> MCU0_TorqueMax_S/1
  MCU0_TorqueMax_S/1 -> MCU0_TorqueMaxcv/1
  MCU0_TorqueMaxcv/1 -> MCU0_TorqueMax_F/1
  MCU0_EmergShutDown_F/1 -> MCU0_EmergShutDown_Ad/1
  MCU0_EmergShutDown_O/1 -> MCU0_EmergShutDown_Ad/2
  MCU0_EmergShutDown_Ad/1 -> MCU0_EmergShutDown_sat/1
  MCU0_EmergShutDown_sat/1 -> MCU0_EmergShutDown_Out/1
  Demux/1 -> MCU0_ControlMode_Sub/1(In1), MCU0_WorkStatus_Sub/1(In1), MCU0_GearStatus_Sub/1(In1), MCU0_HighVol_Sub/1(In1), MCU0_ShutDowAllow_Sub/1(In1), MCU0_EmergShutDown_Sub/1(In1)
  MCU0_EmergShutDown_Sub/1(Out1) -> MCU0_EmergShutDown_Convert/1
  MCU0_EmergShutDown_Convert/1 -> MCU0_EmergShutDown_L/1
  MCU0_EmergShutDown_L/1 -> MCU0_EmergShutDown_S/1
  MCU0_EmergShutDown_S/1 -> MCU0_EmergShutDowncv/1
  MCU0_EmergShutDowncv/1 -> MCU0_EmergShutDown_F/1
  MCU0_ShutDowAllow_F/1 -> MCU0_ShutDowAllow_Ad/1
  MCU0_ShutDowAllow_O/1 -> MCU0_ShutDowAllow_Ad/2
  MCU0_ShutDowAllow_Ad/1 -> MCU0_ShutDowAllow_sat/1
  MCU0_ShutDowAllow_sat/1 -> MCU0_ShutDowAllow_Out/1
  MCU0_ShutDowAllow_Sub/1(Out1) -> MCU0_ShutDowAllow_Convert/1
  MCU0_ShutDowAllow_Convert/1 -> MCU0_ShutDowAllow_L/1
  MCU0_ShutDowAllow_L/1 -> MCU0_ShutDowAllow_S/1
  MCU0_ShutDowAllow_S/1 -> MCU0_ShutDowAllowcv/1
  MCU0_ShutDowAllowcv/1 -> MCU0_ShutDowAllow_F/1
  MCU0_HighVol_F/1 -> MCU0_HighVol_Ad/1
  MCU0_HighVol_O/1 -> MCU0_HighVol_Ad/2
  MCU0_HighVol_Ad/1 -> MCU0_HighVol_sat/1
  MCU0_HighVol_sat/1 -> MCU0_HighVol_Out/1
  MCU0_HighVol_Sub/1(Out1) -> MCU0_HighVol_Convert/1
  MCU0_HighVol_Convert/1 -> MCU0_HighVol_L/1
  MCU0_HighVol_L/1 -> MCU0_HighVol_S/1
  MCU0_HighVol_S/1 -> MCU0_HighVolcv/1
  MCU0_HighVolcv/1 -> MCU0_HighVol_F/1
  MCU0_LiftCnt_F/1 -> MCU0_LiftCnt_Ad/1
  MCU0_LiftCnt_O/1 -> MCU0_LiftCnt_Ad/2
  MCU0_LiftCnt_Ad/1 -> MCU0_LiftCnt_sat/1
  MCU0_LiftCnt_sat/1 -> MCU0_LiftCnt_Out/1
  Demux/8 -> MCU0_LiftCnt_Sub/1(In1)
  MCU0_LiftCnt_Sub/1(Out1) -> MCU0_LiftCnt_Convert/1
  MCU0_LiftCnt_Convert/1 -> MCU0_LiftCnt_L/1
  MCU0_LiftCnt_L/1 -> MCU0_LiftCnt_S/1
  MCU0_LiftCnt_S/1 -> MCU0_LiftCntcv/1
  MCU0_LiftCntcv/1 -> MCU0_LiftCnt_F/1
  MCU0_TorqueFdk_F/1 -> MCU0_TorqueFdk_Ad/1
  MCU0_TorqueFdk_O/1 -> MCU0_TorqueFdk_Ad/2
  MCU0_TorqueFdk_Ad/1 -> MCU0_TorqueFdk_sat/1
  MCU0_TorqueFdk_sat/1 -> MCU0_TorqueFdk_Out/1
  Demux/4 -> MCU0_TorqueFdkinput4_P/1
  MCU0_TorqueFdkinput4_C/1 -> MCU0_TorqueFdkinput4_P/2
  MCU0_TorqueFdkinput4_P/1 -> MCU0_TorqueFdkinput4_Ad/1
  Demux/5 -> MCU0_TorqueFdkinput4_Ad/2
  MCU0_TorqueFdkinput4_Ad/1 -> MCU0_TorqueFdk_Sub/1(In1)
  MCU0_TorqueFdk_Sub/1(Out1) -> MCU0_TorqueFdk_Convert/1
  MCU0_TorqueFdk_Convert/1 -> MCU0_TorqueFdk_L/1
  MCU0_TorqueFdk_L/1 -> MCU0_TorqueFdk_S/1
  MCU0_TorqueFdk_S/1 -> MCU0_TorqueFdkcv/1
  MCU0_TorqueFdkcv/1 -> MCU0_TorqueFdk_F/1
  MCU0_SpeedFdk_F/1 -> MCU0_SpeedFdk_Ad/1
  MCU0_SpeedFdk_O/1 -> MCU0_SpeedFdk_Ad/2
  MCU0_SpeedFdk_Ad/1 -> MCU0_SpeedFdk_sat/1
  MCU0_SpeedFdk_sat/1 -> MCU0_SpeedFdk_Out/1
  Demux/2 -> MCU0_SpeedFdkinput2_P/1
  MCU0_SpeedFdkinput2_C/1 -> MCU0_SpeedFdkinput2_P/2
  MCU0_SpeedFdkinput2_P/1 -> MCU0_SpeedFdkinput2_Ad/1
  Demux/3 -> MCU0_SpeedFdkinput2_Ad/2
  MCU0_SpeedFdkinput2_Ad/1 -> MCU0_SpeedFdk_Sub/1(In1)
  MCU0_SpeedFdk_Sub/1(Out1) -> MCU0_SpeedFdk_Convert/1
  MCU0_SpeedFdk_Convert/1 -> MCU0_SpeedFdk_L/1
  MCU0_SpeedFdk_L/1 -> MCU0_SpeedFdk_S/1
  MCU0_SpeedFdk_S/1 -> MCU0_SpeedFdkcv/1
  MCU0_SpeedFdkcv/1 -> MCU0_SpeedFdk_F/1
  MCU0_GearStatus_F/1 -> MCU0_GearStatus_Ad/1
  MCU0_GearStatus_O/1 -> MCU0_GearStatus_Ad/2
  MCU0_GearStatus_Ad/1 -> MCU0_GearStatus_sat/1
  MCU0_GearStatus_sat/1 -> MCU0_GearStatus_Out/1
  MCU0_GearStatus_Sub/1(Out1) -> MCU0_GearStatus_Convert/1
  MCU0_GearStatus_Convert/1 -> MCU0_GearStatus_L/1
  MCU0_GearStatus_L/1 -> MCU0_GearStatus_S/1
  MCU0_GearStatus_S/1 -> MCU0_GearStatuscv/1
  MCU0_GearStatuscv/1 -> MCU0_GearStatus_F/1
  MCU0_ControlMode_F/1 -> MCU0_ControlMode_Ad/1
  MCU0_ControlMode_O/1 -> MCU0_ControlMode_Ad/2
  MCU0_ControlMode_Ad/1 -> MCU0_ControlMode_sat/1
  MCU0_ControlMode_sat/1 -> MCU0_ControlMode_Out/1
  MCU0_ControlMode_Sub/1(Out1) -> MCU0_ControlMode_Convert/1
  MCU0_ControlMode_Convert/1 -> MCU0_ControlMode_L/1
  MCU0_ControlMode_L/1 -> MCU0_ControlMode_S/1
  MCU0_ControlMode_S/1 -> MCU0_ControlModecv/1
  MCU0_ControlModecv/1 -> MCU0_ControlMode_F/1
  MCU0_WorkStatus_F/1 -> MCU0_WorkStatus_Ad/1
  MCU0_WorkStatus_O/1 -> MCU0_WorkStatus_Ad/2
  MCU0_WorkStatus_Ad/1 -> MCU0_WorkStatus_sat/1
  MCU0_WorkStatus_sat/1 -> MCU0_WorkStatus_Out/1
  MCU0_WorkStatus_Sub/1(Out1) -> MCU0_WorkStatus_Convert/1
  MCU0_WorkStatus_Convert/1 -> MCU0_WorkStatus_L/1
  MCU0_WorkStatus_L/1 -> MCU0_WorkStatus_S/1
  MCU0_WorkStatus_S/1 -> MCU0_WorkStatuscv/1
  MCU0_WorkStatuscv/1 -> MCU0_WorkStatus_F/1
  input/1 -> Demux/1

== system six_plus_six_AcmsteeringV09_main/Data_input/MCU1/MCU1 ==
  input : Inport
  Enable : EnablePort
  Demux : Demux  Outputs=8
  MCU1_ControlTemp_Ad : Sum
  MCU1_ControlTemp_Convert : DataTypeConversion  OutDataTypeStr=uint32
  MCU1_ControlTemp_F : Gain
  MCU1_ControlTemp_L : simulink/Logic and Bit Operations/Bitwise Operator  logicop=AND  UseBitMask=on  BitMask=255  BitMaskRealWorld=Stored Integer
  MCU1_ControlTemp_O : Constant  Value=-40  OutDataTypeStr=single
  MCU1_ControlTemp_S : ArithShift
  MCU1_ControlTemp_Sub : Subsystem
  MCU1_ControlTemp_sat : Saturate  UpperLimit=215  LowerLimit=-40
  MCU1_ControlTempcv : DataTypeConversion
  MCU1_Idc_Ad : Sum
  MCU1_Idc_Convert : DataTypeConversion  OutDataTypeStr=uint32
  MCU1_Idc_F : Gain  Gain=0.1
  MCU1_Idc_L : simulink/Logic and Bit Operations/Bitwise Operator  logicop=AND  UseBitMask=on  BitMask=65535  BitMaskRealWorld=Stored Integer
  MCU1_Idc_O : Constant  Value=-1600  OutDataTypeStr=single
  MCU1_Idc_S : ArithShift
  MCU1_Idc_Sub : Subsystem
  MCU1_Idc_sat : Saturate  UpperLimit=1600  LowerLimit=-1600
  MCU1_Idccv : DataTypeConversion
  MCU1_Idcinput3_Ad : Sum
  MCU1_Idcinput3_C : Constant  Value=256
  MCU1_Idcinput3_P : Product
  MCU1_MotorTemp_Ad : Sum
  MCU1_MotorTemp_Convert : DataTypeConversion  OutDataTypeStr=uint32
  MCU1_MotorTemp_F : Gain
  MCU1_MotorTemp_L : simulink/Logic and Bit Operations/Bitwise Operator  logicop=AND  UseBitMask=on  BitMask=255  BitMaskRealWorld=Stored Integer
  MCU1_MotorTemp_O : Constant  Value=-40  OutDataTypeStr=single
  MCU1_MotorTemp_S : ArithShift
  MCU1_MotorTemp_Sub : Subsystem
  MCU1_MotorTemp_sat : Saturate  UpperLimit=215  LowerLimit=-40
  MCU1_MotorTempcv : DataTypeConversion
  MCU1_PowerFdk_Ad : Sum
  MCU1_PowerFdk_Convert : DataTypeConversion  OutDataTypeStr=uint32
  MCU1_PowerFdk_F : Gain
  MCU1_PowerFdk_L : simulink/Logic and Bit Operations/Bitwise Operator  logicop=AND  UseBitMask=on  BitMask=65535  BitMaskRealWorld=Stored Integer
  MCU1_PowerFdk_O : Constant  Value=0  OutDataTypeStr=single
  MCU1_PowerFdk_S : ArithShift
  MCU1_PowerFdk_Sub : Subsystem
  MCU1_PowerFdk_sat : Saturate  UpperLimit=65535  LowerLimit=0
  MCU1_PowerFdkcv : DataTypeConversion
  MCU1_PowerFdkinput5_Ad : Sum
  MCU1_PowerFdkinput5_C : Constant  Value=256
  MCU1_PowerFdkinput5_P : Product
  MCU1_Udc_Ad : Sum
  MCU1_Udc_Convert : DataTypeConversion  OutDataTypeStr=uint32
  MCU1_Udc_F : Gain  Gain=0.1
  MCU1_Udc_L : simulink/Logic and Bit Operations/Bitwise Operator  logicop=AND  UseBitMask=on  BitMask=65535  BitMaskRealWorld=Stored Integer
  MCU1_Udc_O : Constant  Value=0  OutDataTypeStr=single
  MCU1_Udc_S : ArithShift
  MCU1_Udc_Sub : Subsystem
  MCU1_Udc_sat : Saturate  UpperLimit=1000  LowerLimit=0
  MCU1_Udccv : DataTypeConversion
  MCU1_Udcinput1_Ad : Sum
  MCU1_Udcinput1_C : Constant  Value=256
  MCU1_Udcinput1_P : Product
  MCU1_ControlTemp_Out : Outport
  MCU1_MotorTemp_Out : Outport  Port=2
  MCU1_PowerFdk_Out : Outport  Port=3
  MCU1_Idc_Out : Outport  Port=4
  MCU1_Udc_Out : Outport  Port=5
  wires:
  MCU1_ControlTemp_F/1 -> MCU1_ControlTemp_Ad/1
  MCU1_ControlTemp_O/1 -> MCU1_ControlTemp_Ad/2
  MCU1_ControlTemp_Ad/1 -> MCU1_ControlTemp_sat/1
  MCU1_ControlTemp_sat/1 -> MCU1_ControlTemp_Out/1
  Demux/8 -> MCU1_ControlTemp_Sub/1(In1)
  MCU1_ControlTemp_Sub/1(Out1) -> MCU1_ControlTemp_Convert/1
  MCU1_ControlTemp_Convert/1 -> MCU1_ControlTemp_L/1
  MCU1_ControlTemp_L/1 -> MCU1_ControlTemp_S/1
  MCU1_ControlTemp_S/1 -> MCU1_ControlTempcv/1
  MCU1_ControlTempcv/1 -> MCU1_ControlTemp_F/1
  MCU1_MotorTemp_F/1 -> MCU1_MotorTemp_Ad/1
  MCU1_MotorTemp_O/1 -> MCU1_MotorTemp_Ad/2
  MCU1_MotorTemp_Ad/1 -> MCU1_MotorTemp_sat/1
  MCU1_MotorTemp_sat/1 -> MCU1_MotorTemp_Out/1
  Demux/7 -> MCU1_MotorTemp_Sub/1(In1)
  MCU1_MotorTemp_Sub/1(Out1) -> MCU1_MotorTemp_Convert/1
  MCU1_MotorTemp_Convert/1 -> MCU1_MotorTemp_L/1
  MCU1_MotorTemp_L/1 -> MCU1_MotorTemp_S/1
  MCU1_MotorTemp_S/1 -> MCU1_MotorTempcv/1
  MCU1_MotorTempcv/1 -> MCU1_MotorTemp_F/1
  MCU1_PowerFdk_F/1 -> MCU1_PowerFdk_Ad/1
  MCU1_PowerFdk_O/1 -> MCU1_PowerFdk_Ad/2
  MCU1_PowerFdk_Ad/1 -> MCU1_PowerFdk_sat/1
  MCU1_PowerFdk_sat/1 -> MCU1_PowerFdk_Out/1
  Demux/5 -> MCU1_PowerFdkinput5_P/1
  MCU1_PowerFdkinput5_C/1 -> MCU1_PowerFdkinput5_P/2
  MCU1_PowerFdkinput5_P/1 -> MCU1_PowerFdkinput5_Ad/1
  Demux/6 -> MCU1_PowerFdkinput5_Ad/2
  MCU1_PowerFdkinput5_Ad/1 -> MCU1_PowerFdk_Sub/1(In1)
  MCU1_PowerFdk_Sub/1(Out1) -> MCU1_PowerFdk_Convert/1
  MCU1_PowerFdk_Convert/1 -> MCU1_PowerFdk_L/1
  MCU1_PowerFdk_L/1 -> MCU1_PowerFdk_S/1
  MCU1_PowerFdk_S/1 -> MCU1_PowerFdkcv/1
  MCU1_PowerFdkcv/1 -> MCU1_PowerFdk_F/1
  MCU1_Idc_F/1 -> MCU1_Idc_Ad/1
  MCU1_Idc_O/1 -> MCU1_Idc_Ad/2
  MCU1_Idc_Ad/1 -> MCU1_Idc_sat/1
  MCU1_Idc_sat/1 -> MCU1_Idc_Out/1
  Demux/3 -> MCU1_Idcinput3_P/1
  MCU1_Idcinput3_C/1 -> MCU1_Idcinput3_P/2
  MCU1_Idcinput3_P/1 -> MCU1_Idcinput3_Ad/1
  Demux/4 -> MCU1_Idcinput3_Ad/2
  MCU1_Idcinput3_Ad/1 -> MCU1_Idc_Sub/1(In1)
  MCU1_Idc_Sub/1(Out1) -> MCU1_Idc_Convert/1
  MCU1_Idc_Convert/1 -> MCU1_Idc_L/1
  MCU1_Idc_L/1 -> MCU1_Idc_S/1
  MCU1_Idc_S/1 -> MCU1_Idccv/1
  MCU1_Idccv/1 -> MCU1_Idc_F/1
  MCU1_Udc_F/1 -> MCU1_Udc_Ad/1
  MCU1_Udc_O/1 -> MCU1_Udc_Ad/2
  MCU1_Udc_Ad/1 -> MCU1_Udc_sat/1
  MCU1_Udc_sat/1 -> MCU1_Udc_Out/1
  Demux/1 -> MCU1_Udcinput1_P/1
  MCU1_Udcinput1_C/1 -> MCU1_Udcinput1_P/2
  MCU1_Udcinput1_P/1 -> MCU1_Udcinput1_Ad/1
  Demux/2 -> MCU1_Udcinput1_Ad/2
  MCU1_Udcinput1_Ad/1 -> MCU1_Udc_Sub/1(In1)
  MCU1_Udc_Sub/1(Out1) -> MCU1_Udc_Convert/1
  MCU1_Udc_Convert/1 -> MCU1_Udc_L/1
  MCU1_Udc_L/1 -> MCU1_Udc_S/1
  MCU1_Udc_S/1 -> MCU1_Udccv/1
  MCU1_Udccv/1 -> MCU1_Udc_F/1
  input/1 -> Demux/1

== system six_plus_six_AcmsteeringV09_main/Data_input/MCU1_1/MCU1 ==
  input : Inport
  Enable : EnablePort
  Demux : Demux  Outputs=8
  MCU1_ControlTemp_Ad : Sum
  MCU1_ControlTemp_Convert : DataTypeConversion  OutDataTypeStr=uint32
  MCU1_ControlTemp_F : Gain
  MCU1_ControlTemp_L : simulink/Logic and Bit Operations/Bitwise Operator  logicop=AND  UseBitMask=on  BitMask=255  BitMaskRealWorld=Stored Integer
  MCU1_ControlTemp_O : Constant  Value=-40  OutDataTypeStr=single
  MCU1_ControlTemp_S : ArithShift
  MCU1_ControlTemp_Sub : Subsystem
  MCU1_ControlTemp_sat : Saturate  UpperLimit=215  LowerLimit=-40
  MCU1_ControlTempcv : DataTypeConversion
  MCU1_Idc_Ad : Sum
  MCU1_Idc_Convert : DataTypeConversion  OutDataTypeStr=uint32
  MCU1_Idc_F : Gain  Gain=0.1
  MCU1_Idc_L : simulink/Logic and Bit Operations/Bitwise Operator  logicop=AND  UseBitMask=on  BitMask=65535  BitMaskRealWorld=Stored Integer
  MCU1_Idc_O : Constant  Value=-1600  OutDataTypeStr=single
  MCU1_Idc_S : ArithShift
  MCU1_Idc_Sub : Subsystem
  MCU1_Idc_sat : Saturate  UpperLimit=1600  LowerLimit=-1600
  MCU1_Idccv : DataTypeConversion
  MCU1_Idcinput3_Ad : Sum
  MCU1_Idcinput3_C : Constant  Value=256
  MCU1_Idcinput3_P : Product
  MCU1_MotorTemp_Ad : Sum
  MCU1_MotorTemp_Convert : DataTypeConversion  OutDataTypeStr=uint32
  MCU1_MotorTemp_F : Gain
  MCU1_MotorTemp_L : simulink/Logic and Bit Operations/Bitwise Operator  logicop=AND  UseBitMask=on  BitMask=255  BitMaskRealWorld=Stored Integer
  MCU1_MotorTemp_O : Constant  Value=-40  OutDataTypeStr=single
  MCU1_MotorTemp_S : ArithShift
  MCU1_MotorTemp_Sub : Subsystem
  MCU1_MotorTemp_sat : Saturate  UpperLimit=215  LowerLimit=-40
  MCU1_MotorTempcv : DataTypeConversion
  MCU1_PowerFdk_Ad : Sum
  MCU1_PowerFdk_Convert : DataTypeConversion  OutDataTypeStr=uint32
  MCU1_PowerFdk_F : Gain
  MCU1_PowerFdk_L : simulink/Logic and Bit Operations/Bitwise Operator  logicop=AND  UseBitMask=on  BitMask=65535  BitMaskRealWorld=Stored Integer
  MCU1_PowerFdk_O : Constant  Value=0  OutDataTypeStr=single
  MCU1_PowerFdk_S : ArithShift
  MCU1_PowerFdk_Sub : Subsystem
  MCU1_PowerFdk_sat : Saturate  UpperLimit=65535  LowerLimit=0
  MCU1_PowerFdkcv : DataTypeConversion
  MCU1_PowerFdkinput5_Ad : Sum
  MCU1_PowerFdkinput5_C : Constant  Value=256
  MCU1_PowerFdkinput5_P : Product
  MCU1_Udc_Ad : Sum
  MCU1_Udc_Convert : DataTypeConversion  OutDataTypeStr=uint32
  MCU1_Udc_F : Gain  Gain=0.1
  MCU1_Udc_L : simulink/Logic and Bit Operations/Bitwise Operator  logicop=AND  UseBitMask=on  BitMask=65535  BitMaskRealWorld=Stored Integer
  MCU1_Udc_O : Constant  Value=0  OutDataTypeStr=single
  MCU1_Udc_S : ArithShift
  MCU1_Udc_Sub : Subsystem
  MCU1_Udc_sat : Saturate  UpperLimit=1000  LowerLimit=0
  MCU1_Udccv : DataTypeConversion
  MCU1_Udcinput1_Ad : Sum
  MCU1_Udcinput1_C : Constant  Value=256
  MCU1_Udcinput1_P : Product
  MCU1_ControlTemp_Out : Outport
  MCU1_MotorTemp_Out : Outport  Port=2
  MCU1_PowerFdk_Out : Outport  Port=3
  MCU1_Idc_Out : Outport  Port=4
  MCU1_Udc_Out : Outport  Port=5
  wires:
  MCU1_ControlTemp_F/1 -> MCU1_ControlTemp_Ad/1
  MCU1_ControlTemp_O/1 -> MCU1_ControlTemp_Ad/2
  MCU1_ControlTemp_Ad/1 -> MCU1_ControlTemp_sat/1
  MCU1_ControlTemp_sat/1 -> MCU1_ControlTemp_Out/1
  Demux/8 -> MCU1_ControlTemp_Sub/1(In1)
  MCU1_ControlTemp_Sub/1(Out1) -> MCU1_ControlTemp_Convert/1
  MCU1_ControlTemp_Convert/1 -> MCU1_ControlTemp_L/1
  MCU1_ControlTemp_L/1 -> MCU1_ControlTemp_S/1
  MCU1_ControlTemp_S/1 -> MCU1_ControlTempcv/1
  MCU1_ControlTempcv/1 -> MCU1_ControlTemp_F/1
  MCU1_MotorTemp_F/1 -> MCU1_MotorTemp_Ad/1
  MCU1_MotorTemp_O/1 -> MCU1_MotorTemp_Ad/2
  MCU1_MotorTemp_Ad/1 -> MCU1_MotorTemp_sat/1
  MCU1_MotorTemp_sat/1 -> MCU1_MotorTemp_Out/1
  Demux/7 -> MCU1_MotorTemp_Sub/1(In1)
  MCU1_MotorTemp_Sub/1(Out1) -> MCU1_MotorTemp_Convert/1
  MCU1_MotorTemp_Convert/1 -> MCU1_MotorTemp_L/1
  MCU1_MotorTemp_L/1 -> MCU1_MotorTemp_S/1
  MCU1_MotorTemp_S/1 -> MCU1_MotorTempcv/1
  MCU1_MotorTempcv/1 -> MCU1_MotorTemp_F/1
  MCU1_PowerFdk_F/1 -> MCU1_PowerFdk_Ad/1
  MCU1_PowerFdk_O/1 -> MCU1_PowerFdk_Ad/2
  MCU1_PowerFdk_Ad/1 -> MCU1_PowerFdk_sat/1
  MCU1_PowerFdk_sat/1 -> MCU1_PowerFdk_Out/1
  Demux/5 -> MCU1_PowerFdkinput5_P/1
  MCU1_PowerFdkinput5_C/1 -> MCU1_PowerFdkinput5_P/2
  MCU1_PowerFdkinput5_P/1 -> MCU1_PowerFdkinput5_Ad/1
  Demux/6 -> MCU1_PowerFdkinput5_Ad/2
  MCU1_PowerFdkinput5_Ad/1 -> MCU1_PowerFdk_Sub/1(In1)
  MCU1_PowerFdk_Sub/1(Out1) -> MCU1_PowerFdk_Convert/1
  MCU1_PowerFdk_Convert/1 -> MCU1_PowerFdk_L/1
  MCU1_PowerFdk_L/1 -> MCU1_PowerFdk_S/1
  MCU1_PowerFdk_S/1 -> MCU1_PowerFdkcv/1
  MCU1_PowerFdkcv/1 -> MCU1_PowerFdk_F/1
  MCU1_Idc_F/1 -> MCU1_Idc_Ad/1
  MCU1_Idc_O/1 -> MCU1_Idc_Ad/2
  MCU1_Idc_Ad/1 -> MCU1_Idc_sat/1
  MCU1_Idc_sat/1 -> MCU1_Idc_Out/1
  Demux/3 -> MCU1_Idcinput3_P/1
  MCU1_Idcinput3_C/1 -> MCU1_Idcinput3_P/2
  MCU1_Idcinput3_P/1 -> MCU1_Idcinput3_Ad/1
  Demux/4 -> MCU1_Idcinput3_Ad/2
  MCU1_Idcinput3_Ad/1 -> MCU1_Idc_Sub/1(In1)
  MCU1_Idc_Sub/1(Out1) -> MCU1_Idc_Convert/1
  MCU1_Idc_Convert/1 -> MCU1_Idc_L/1
  MCU1_Idc_L/1 -> MCU1_Idc_S/1
  MCU1_Idc_S/1 -> MCU1_Idccv/1
  MCU1_Idccv/1 -> MCU1_Idc_F/1
  MCU1_Udc_F/1 -> MCU1_Udc_Ad/1
  MCU1_Udc_O/1 -> MCU1_Udc_Ad/2
  MCU1_Udc_Ad/1 -> MCU1_Udc_sat/1
  MCU1_Udc_sat/1 -> MCU1_Udc_Out/1
  Demux/1 -> MCU1_Udcinput1_P/1
  MCU1_Udcinput1_C/1 -> MCU1_Udcinput1_P/2
  MCU1_Udcinput1_P/1 -> MCU1_Udcinput1_Ad/1
  Demux/2 -> MCU1_Udcinput1_Ad/2
  MCU1_Udcinput1_Ad/1 -> MCU1_Udc_Sub/1(In1)
  MCU1_Udc_Sub/1(Out1) -> MCU1_Udc_Convert/1
  MCU1_Udc_Convert/1 -> MCU1_Udc_L/1
  MCU1_Udc_L/1 -> MCU1_Udc_S/1
  MCU1_Udc_S/1 -> MCU1_Udccv/1
  MCU1_Udccv/1 -> MCU1_Udc_F/1
  input/1 -> Demux/1

== system six_plus_six_AcmsteeringV09_main/Data_input/MCU1_2/MCU1 ==
  input : Inport
  Enable : EnablePort
  Demux : Demux  Outputs=8
  MCU1_ControlTemp_Ad : Sum
  MCU1_ControlTemp_Convert : DataTypeConversion  OutDataTypeStr=uint32
  MCU1_ControlTemp_F : Gain
  MCU1_ControlTemp_L : simulink/Logic and Bit Operations/Bitwise Operator  logicop=AND  UseBitMask=on  BitMask=255  BitMaskRealWorld=Stored Integer
  MCU1_ControlTemp_O : Constant  Value=-40  OutDataTypeStr=single
  MCU1_ControlTemp_S : ArithShift
  MCU1_ControlTemp_Sub : Subsystem
  MCU1_ControlTemp_sat : Saturate  UpperLimit=215  LowerLimit=-40
  MCU1_ControlTempcv : DataTypeConversion
  MCU1_Idc_Ad : Sum
  MCU1_Idc_Convert : DataTypeConversion  OutDataTypeStr=uint32
  MCU1_Idc_F : Gain  Gain=0.1
  MCU1_Idc_L : simulink/Logic and Bit Operations/Bitwise Operator  logicop=AND  UseBitMask=on  BitMask=65535  BitMaskRealWorld=Stored Integer
  MCU1_Idc_O : Constant  Value=-1600  OutDataTypeStr=single
  MCU1_Idc_S : ArithShift
  MCU1_Idc_Sub : Subsystem
  MCU1_Idc_sat : Saturate  UpperLimit=1600  LowerLimit=-1600
  MCU1_Idccv : DataTypeConversion
  MCU1_Idcinput3_Ad : Sum
  MCU1_Idcinput3_C : Constant  Value=256
  MCU1_Idcinput3_P : Product
  MCU1_MotorTemp_Ad : Sum
  MCU1_MotorTemp_Convert : DataTypeConversion  OutDataTypeStr=uint32
  MCU1_MotorTemp_F : Gain
  MCU1_MotorTemp_L : simulink/Logic and Bit Operations/Bitwise Operator  logicop=AND  UseBitMask=on  BitMask=255  BitMaskRealWorld=Stored Integer
  MCU1_MotorTemp_O : Constant  Value=-40  OutDataTypeStr=single
  MCU1_MotorTemp_S : ArithShift
  MCU1_MotorTemp_Sub : Subsystem
  MCU1_MotorTemp_sat : Saturate  UpperLimit=215  LowerLimit=-40
  MCU1_MotorTempcv : DataTypeConversion
  MCU1_PowerFdk_Ad : Sum
  MCU1_PowerFdk_Convert : DataTypeConversion  OutDataTypeStr=uint32
  MCU1_PowerFdk_F : Gain
  MCU1_PowerFdk_L : simulink/Logic and Bit Operations/Bitwise Operator  logicop=AND  UseBitMask=on  BitMask=65535  BitMaskRealWorld=Stored Integer
  MCU1_PowerFdk_O : Constant  Value=0  OutDataTypeStr=single
  MCU1_PowerFdk_S : ArithShift
  MCU1_PowerFdk_Sub : Subsystem
  MCU1_PowerFdk_sat : Saturate  UpperLimit=65535  LowerLimit=0
  MCU1_PowerFdkcv : DataTypeConversion
  MCU1_PowerFdkinput5_Ad : Sum
  MCU1_PowerFdkinput5_C : Constant  Value=256
  MCU1_PowerFdkinput5_P : Product
  MCU1_Udc_Ad : Sum
  MCU1_Udc_Convert : DataTypeConversion  OutDataTypeStr=uint32
  MCU1_Udc_F : Gain  Gain=0.1
  MCU1_Udc_L : simulink/Logic and Bit Operations/Bitwise Operator  logicop=AND  UseBitMask=on  BitMask=65535  BitMaskRealWorld=Stored Integer
  MCU1_Udc_O : Constant  Value=0  OutDataTypeStr=single
  MCU1_Udc_S : ArithShift
  MCU1_Udc_Sub : Subsystem
  MCU1_Udc_sat : Saturate  UpperLimit=1000  LowerLimit=0
  MCU1_Udccv : DataTypeConversion
  MCU1_Udcinput1_Ad : Sum
  MCU1_Udcinput1_C : Constant  Value=256
  MCU1_Udcinput1_P : Product
  MCU1_ControlTemp_Out : Outport
  MCU1_MotorTemp_Out : Outport  Port=2
  MCU1_PowerFdk_Out : Outport  Port=3
  MCU1_Idc_Out : Outport  Port=4
  MCU1_Udc_Out : Outport  Port=5
  wires:
  MCU1_ControlTemp_F/1 -> MCU1_ControlTemp_Ad/1
  MCU1_ControlTemp_O/1 -> MCU1_ControlTemp_Ad/2
  MCU1_ControlTemp_Ad/1 -> MCU1_ControlTemp_sat/1
  MCU1_ControlTemp_sat/1 -> MCU1_ControlTemp_Out/1
  Demux/8 -> MCU1_ControlTemp_Sub/1(In1)
  MCU1_ControlTemp_Sub/1(Out1) -> MCU1_ControlTemp_Convert/1
  MCU1_ControlTemp_Convert/1 -> MCU1_ControlTemp_L/1
  MCU1_ControlTemp_L/1 -> MCU1_ControlTemp_S/1
  MCU1_ControlTemp_S/1 -> MCU1_ControlTempcv/1
  MCU1_ControlTempcv/1 -> MCU1_ControlTemp_F/1
  MCU1_MotorTemp_F/1 -> MCU1_MotorTemp_Ad/1
  MCU1_MotorTemp_O/1 -> MCU1_MotorTemp_Ad/2
  MCU1_MotorTemp_Ad/1 -> MCU1_MotorTemp_sat/1
  MCU1_MotorTemp_sat/1 -> MCU1_MotorTemp_Out/1
  Demux/7 -> MCU1_MotorTemp_Sub/1(In1)
  MCU1_MotorTemp_Sub/1(Out1) -> MCU1_MotorTemp_Convert/1
  MCU1_MotorTemp_Convert/1 -> MCU1_MotorTemp_L/1
  MCU1_MotorTemp_L/1 -> MCU1_MotorTemp_S/1
  MCU1_MotorTemp_S/1 -> MCU1_MotorTempcv/1
  MCU1_MotorTempcv/1 -> MCU1_MotorTemp_F/1
  MCU1_PowerFdk_F/1 -> MCU1_PowerFdk_Ad/1
  MCU1_PowerFdk_O/1 -> MCU1_PowerFdk_Ad/2
  MCU1_PowerFdk_Ad/1 -> MCU1_PowerFdk_sat/1
  MCU1_PowerFdk_sat/1 -> MCU1_PowerFdk_Out/1
  Demux/5 -> MCU1_PowerFdkinput5_P/1
  MCU1_PowerFdkinput5_C/1 -> MCU1_PowerFdkinput5_P/2
  MCU1_PowerFdkinput5_P/1 -> MCU1_PowerFdkinput5_Ad/1
  Demux/6 -> MCU1_PowerFdkinput5_Ad/2
  MCU1_PowerFdkinput5_Ad/1 -> MCU1_PowerFdk_Sub/1(In1)
  MCU1_PowerFdk_Sub/1(Out1) -> MCU1_PowerFdk_Convert/1
  MCU1_PowerFdk_Convert/1 -> MCU1_PowerFdk_L/1
  MCU1_PowerFdk_L/1 -> MCU1_PowerFdk_S/1
  MCU1_PowerFdk_S/1 -> MCU1_PowerFdkcv/1
  MCU1_PowerFdkcv/1 -> MCU1_PowerFdk_F/1
  MCU1_Idc_F/1 -> MCU1_Idc_Ad/1
  MCU1_Idc_O/1 -> MCU1_Idc_Ad/2
  MCU1_Idc_Ad/1 -> MCU1_Idc_sat/1
  MCU1_Idc_sat/1 -> MCU1_Idc_Out/1
  Demux/3 -> MCU1_Idcinput3_P/1
  MCU1_Idcinput3_C/1 -> MCU1_Idcinput3_P/2
  MCU1_Idcinput3_P/1 -> MCU1_Idcinput3_Ad/1
  Demux/4 -> MCU1_Idcinput3_Ad/2
  MCU1_Idcinput3_Ad/1 -> MCU1_Idc_Sub/1(In1)
  MCU1_Idc_Sub/1(Out1) -> MCU1_Idc_Convert/1
  MCU1_Idc_Convert/1 -> MCU1_Idc_L/1
  MCU1_Idc_L/1 -> MCU1_Idc_S/1
  MCU1_Idc_S/1 -> MCU1_Idccv/1
  MCU1_Idccv/1 -> MCU1_Idc_F/1
  MCU1_Udc_F/1 -> MCU1_Udc_Ad/1
  MCU1_Udc_O/1 -> MCU1_Udc_Ad/2
  MCU1_Udc_Ad/1 -> MCU1_Udc_sat/1
  MCU1_Udc_sat/1 -> MCU1_Udc_Out/1
  Demux/1 -> MCU1_Udcinput1_P/1
  MCU1_Udcinput1_C/1 -> MCU1_Udcinput1_P/2
  MCU1_Udcinput1_P/1 -> MCU1_Udcinput1_Ad/1
  Demux/2 -> MCU1_Udcinput1_Ad/2
  MCU1_Udcinput1_Ad/1 -> MCU1_Udc_Sub/1(In1)
  MCU1_Udc_Sub/1(Out1) -> MCU1_Udc_Convert/1
  MCU1_Udc_Convert/1 -> MCU1_Udc_L/1
  MCU1_Udc_L/1 -> MCU1_Udc_S/1
  MCU1_Udc_S/1 -> MCU1_Udccv/1
  MCU1_Udccv/1 -> MCU1_Udc_F/1
  input/1 -> Demux/1
